simulink model "H_inf_pos_control"  (R2024a)
settings: Solver=VariableStepAuto  StartTime=0.0  StopTime=20  MaxStep=0.1  RelTol=1e-3
values from neighbouring files (symbols this model uses):
  k = 0.5    [H_inf_pos_control_calc.m]
  K_tf = tf(K{i})    [H_inf_pos_control_calc.m]
  m = 10    [H_inf_pos_control_calc.m]
libraries: simulink x1
settings Model: Creator=berto  LastModifiedBy=berto

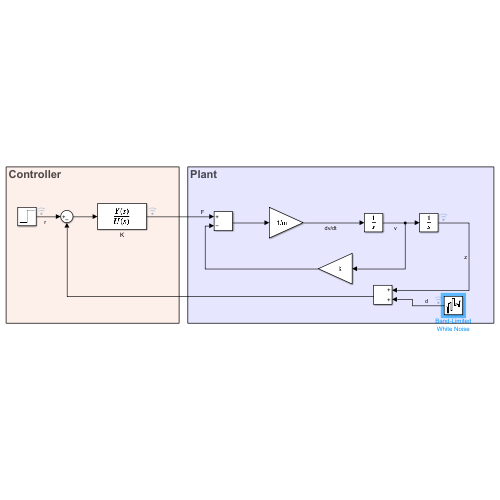
[thumbnail: Simulink's stored preview of the top-level diagram]
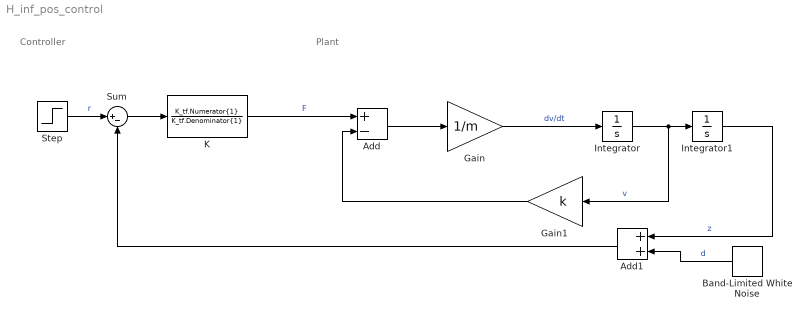
== system H_inf_pos_control ==
  note: Controller
  note: Plant
  Add : Sum  Inputs=+-
  Add1 : Sum
  Band-Limited White Noise : simulink/Sources/Band-Limited White Noise  Cov=[0.0001]  Ts=0.1  seed=[23341]
  Gain : Gain  Gain=1/m
  Gain1 : Gain  Gain=k
  Integrator : Integrator
  Integrator1 : Integrator
  K : TransferFcn  Numerator=K_tf.Numerator{1}  Denominator=K_tf.Denominator{1}
  Step : Step  SampleTime=0
  Sum : Sum  Inputs=|+-
  wires:
  K/1 -> Add/1  "F"
  Step/1 -> Sum/1  "r"
  Sum/1 -> K/1
  Integrator1/1 -> Add1/1  "z"
  Add/1 -> Gain/1
  Gain/1 -> Integrator/1  "dv/dt"
  Integrator/1 -> Gain1/1, Integrator1/1  "v"
  Gain1/1 -> Add/2
  Band-Limited White Noise/1 -> Add1/2  "d"
  Add1/1 -> Sum/2
